simulink model "VentilatorActivity"  (R2024b)
settings: Solver=VariableStepAuto  StartTime=0.0  StopTime=10.0  RelTol=1e-3
model workspace (MAT data in the model file):
  HeatCmd = Simulink.Bus
  HeatCmd.Alignment = -1
  HeatCmd.PreserveElementDimensions = 0
  HeatCmd.Elements_internal = Simulink.BusElement
  HeatCmd.Elements_internal.DimensionsMode = 'Fixed'
  HeatCmd.Elements_internal.SamplingMode = 'Sample based'
  HeatCmd.Elements_internal.SampleTime = -1
  HeatCmd.Elements_internal.Name = 'Element'
  HeatCmd.Elements_internal.DataType_internal = 'double'
  HeatCmd.Elements_internal.Complexity = 'real'
  HeatCmd.Elements_internal.Dimensions = 1
  HeatCmd.DataScope = 'Auto'
  HeaterCmd = Simulink.Bus
  HeaterCmd.Alignment = -1
  HeaterCmd.PreserveElementDimensions = 0
  HeaterCmd.DataScope = 'Auto'
  HumidSens = Simulink.Bus
  HumidSens.Alignment = -1
  HumidSens.PreserveElementDimensions = 0
  HumidSens.DataScope = 'Auto'
  init = Simulink.Bus
  init.Alignment = -1
  init.PreserveElementDimensions = 0
  init.DataScope = 'Auto'
settings Model: Creator=ppatel  LastModifiedBy=ppatel

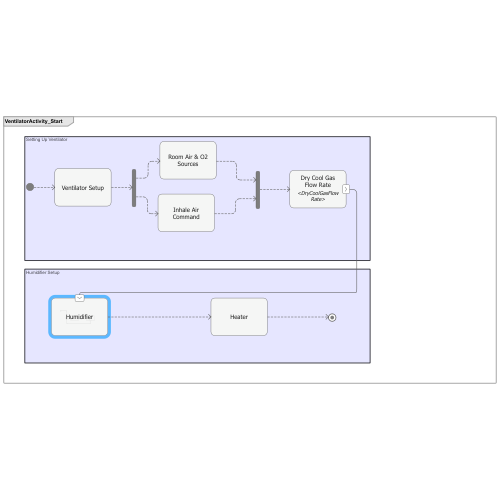
[thumbnail: Simulink's stored preview of the top-level diagram]
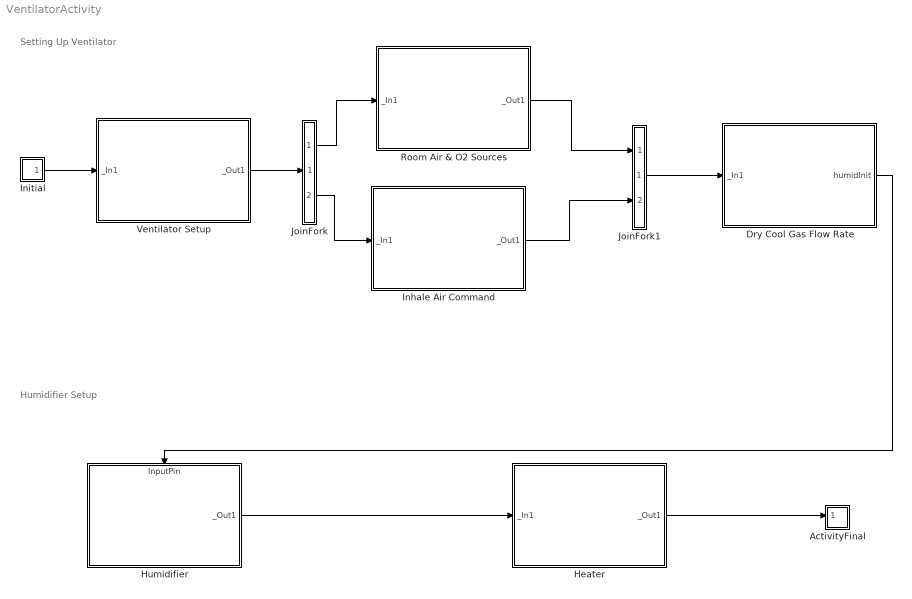
== system VentilatorActivity ==
  note: Humidifier Setup
  note: Setting Up Ventilator
  ActivityFinal : Subsystem
      settings: CopyFcn=set_param(gcbh,'LinkStatus','none');  PortSchema="{\"entries\":[{\"content\":{\"sides\":[{\"content\":{\"connectorIds\":[\"In1\"]},\"type\":\"ConnectorPlacement.EquallySpacedRectSide\",\"uuid\":\"545063dc-4e23-42d6-a986-4c8405208aa1\"},{\"content\":{\"side\":\"RIGHT\"},\"type\":\"ConnectorPlacement.EquallySpacedRectSide\",\"uuid\":\"029392fb-54d3-4ba8-8de1-0e1a97e1bcb4\"},{\"content\":{\"side\":\"TOP\"},\"type\":\"ConnectorPlacement.EquallySpacedRectSide\",\"uuid\":\"54e3c782-8e9d-4642-bf02-641c09921257\"}]},\"type\":\"ConnectorPlacement.EquallySpacedConnector\",\"uuid\":\"f1116680-de99-432f-896c-332f12d99629\"}],\"packageUris\":[\"http://schema.mathworks.com/mf0/Connector/R2020b\"],\"version\":\"1.0\"}"
  Dry Cool Gas Flow Rate : Subsystem
      settings: CopyFcn=set_param(gcbh,'LinkStatus','none');  PortSchema="{\"entries\":[{\"content\":{\"sides\":[{\"content\":{\"connectorIds\":[\"In1\"]},\"type\":\"ConnectorPlacement.EquallySpacedRectSide\",\"uuid\":\"4f1d0bb7-2a97-405d-887b-71e646284e96\"},{\"content\":{\"connectorIds\":[\"Out1\"],\"side\":\"RIGHT\"},\"type\":\"ConnectorPlacement.EquallySpacedRectSide\",\"uuid\":\"0e26442f-68e1-4c32-ac28-bf73737006e5\"},{\"content\":{\"side\":\"TOP\"},\"type\":\"ConnectorPlacement.EquallySpacedRectSide\",\"uuid\":\"07aed82e-d8ef-4f36-9f89-d56db089fe7b\"}]},\"type\":\"ConnectorPlacement.EquallySpacedConnector\",\"uuid\":\"4c88084e-95e1-4023-9a32-ff830e393fdc\"}],\"packageUris\":[\"http://schema.mathworks.com/mf0/Connector/R2020b\"],\"version\":\"1.0\"}"
  Heater : Subsystem
      settings: CopyFcn=set_param(gcbh,'LinkStatus','none');  PortSchema="{\"entries\":[{\"content\":{\"sides\":[{\"content\":{\"connectorIds\":[\"In1\"]},\"type\":\"ConnectorPlacement.EquallySpacedRectSide\",\"uuid\":\"da638e69-4a2c-4548-ace4-820cc1f60a8d\"},{\"content\":{\"connectorIds\":[\"Out1\"],\"side\":\"RIGHT\"},\"type\":\"ConnectorPlacement.EquallySpacedRectSide\",\"uuid\":\"6a8a70e9-7f6e-4f36-a19f-a4054ca44662\"},{\"content\":{\"side\":\"TOP\"},\"type\":\"ConnectorPlacement.EquallySpacedRectSide\",\"uuid\":\"d1e931e2-f76e-4992-8014-0092805a8671\"}]},\"type\":\"ConnectorPlacement.EquallySpacedConnector\",\"uuid\":\"55c0ca13-68f0-475a-9ea9-fab942dd6d78\"}],\"packageUris\":[\"http://schema.mathworks.com/mf0/Connector/R2020b\"],\"version\":\"1.0\"}"
  Humidifier : Subsystem
      settings: CopyFcn=set_param(gcbh,'LinkStatus','none');  PortSchema="{\"entries\":[{\"content\":{\"sides\":[{\"content\":{},\"type\":\"ConnectorPlacement.EquallySpacedRectSide\",\"uuid\":\"da638e69-4a2c-4548-ace4-820cc1f60a8d\"},{\"content\":{\"connectorIds\":[\"Out1\"],\"side\":\"RIGHT\"},\"type\":\"ConnectorPlacement.EquallySpacedRectSide\",\"uuid\":\"6a8a70e9-7f6e-4f36-a19f-a4054ca44662\"},{\"content\":{\"connectorIds\":[\"In1\"],\"side\":\"TOP\"},\"type\":\"ConnectorPlacement.EquallySpacedRectSide\",\"uuid\":\"d1e931e2-f76e-4992-8014-0092805a8671\"}]},\"type\":\"ConnectorPlacement.EquallySpacedConnector\",\"uuid\":\"55c0ca13-68f0-475a-9ea9-fab942dd6d78\"}],\"packageUris\":[\"http://schema.mathworks.com/mf0/Connector/R2020b\"],\"version\":\"1.0\"}"
  Inhale Air Command : Subsystem
      settings: CopyFcn=set_param(gcbh,'LinkStatus','none');  PortSchema="{\"entries\":[{\"content\":{\"sides\":[{\"content\":{\"connectorIds\":[\"In1\"]},\"type\":\"ConnectorPlacement.EquallySpacedRectSide\",\"uuid\":\"da638e69-4a2c-4548-ace4-820cc1f60a8d\"},{\"content\":{\"connectorIds\":[\"Out1\"],\"side\":\"RIGHT\"},\"type\":\"ConnectorPlacement.EquallySpacedRectSide\",\"uuid\":\"6a8a70e9-7f6e-4f36-a19f-a4054ca44662\"},{\"content\":{\"side\":\"TOP\"},\"type\":\"ConnectorPlacement.EquallySpacedRectSide\",\"uuid\":\"d1e931e2-f76e-4992-8014-0092805a8671\"}]},\"type\":\"ConnectorPlacement.EquallySpacedConnector\",\"uuid\":\"55c0ca13-68f0-475a-9ea9-fab942dd6d78\"}],\"packageUris\":[\"http://schema.mathworks.com/mf0/Connector/R2020b\"],\"version\":\"1.0\"}"
  Initial : Subsystem
      settings: CopyFcn=set_param(gcbh,'LinkStatus','none');  PortSchema="{\"entries\":[{\"content\":{\"sides\":[{\"content\":{},\"type\":\"ConnectorPlacement.EquallySpacedRectSide\",\"uuid\":\"da638e69-4a2c-4548-ace4-820cc1f60a8d\"},{\"content\":{\"connectorIds\":[\"Out1\"],\"side\":\"RIGHT\"},\"type\":\"ConnectorPlacement.EquallySpacedRectSide\",\"uuid\":\"6a8a70e9-7f6e-4f36-a19f-a4054ca44662\"},{\"content\":{\"side\":\"TOP\"},\"type\":\"ConnectorPlacement.EquallySpacedRectSide\",\"uuid\":\"d1e931e2-f76e-4992-8014-0092805a8671\"}]},\"type\":\"ConnectorPlacement.EquallySpacedConnector\",\"uuid\":\"55c0ca13-68f0-475a-9ea9-fab942dd6d78\"}],\"packageUris\":[\"http://schema.mathworks.com/mf0/Connector/R2020b\"],\"version\":\"1.0\"}"
  JoinFork : Subsystem
      settings: CopyFcn=set_param(gcbh,'LinkStatus','none');  PortSchema="{\"entries\":[{\"content\":{\"sides\":[{\"content\":{\"connectorIds\":[\"In1\"]},\"type\":\"ConnectorPlacement.EquallySpacedRectSide\",\"uuid\":\"da638e69-4a2c-4548-ace4-820cc1f60a8d\"},{\"content\":{\"connectorIds\":[\"Out1\",\"Out2\"],\"side\":\"RIGHT\"},\"type\":\"ConnectorPlacement.EquallySpacedRectSide\",\"uuid\":\"6a8a70e9-7f6e-4f36-a19f-a4054ca44662\"},{\"content\":{\"side\":\"TOP\"},\"type\":\"ConnectorPlacement.EquallySpacedRectSide\",\"uuid\":\"d1e931e2-f76e-4992-8014-0092805a8671\"}]},\"type\":\"ConnectorPlacement.EquallySpacedConnector\",\"uuid\":\"55c0ca13-68f0-475a-9ea9-fab942dd6d78\"}],\"packageUris\":[\"http://schema.mathworks.com/mf0/Connector/R2020b\"],\"version\":\"1.0\"}"
  JoinFork1 : Subsystem
      settings: CopyFcn=set_param(gcbh,'LinkStatus','none');  PortSchema="{\"entries\":[{\"content\":{\"sides\":[{\"content\":{\"connectorIds\":[\"In1\",\"In2\"]},\"type\":\"ConnectorPlacement.EquallySpacedRectSide\",\"uuid\":\"da638e69-4a2c-4548-ace4-820cc1f60a8d\"},{\"content\":{\"connectorIds\":[\"Out1\"],\"side\":\"RIGHT\"},\"type\":\"ConnectorPlacement.EquallySpacedRectSide\",\"uuid\":\"6a8a70e9-7f6e-4f36-a19f-a4054ca44662\"},{\"content\":{\"side\":\"TOP\"},\"type\":\"ConnectorPlacement.EquallySpacedRectSide\",\"uuid\":\"d1e931e2-f76e-4992-8014-0092805a8671\"}]},\"type\":\"ConnectorPlacement.EquallySpacedConnector\",\"uuid\":\"55c0ca13-68f0-475a-9ea9-fab942dd6d78\"}],\"packageUris\":[\"http://schema.mathworks.com/mf0/Connector/R2020b\"],\"version\":\"1.0\"}"
  Room Air & O2 Sources : Subsystem
      settings: CopyFcn=set_param(gcbh,'LinkStatus','none');  PortSchema="{\"entries\":[{\"content\":{\"sides\":[{\"content\":{\"connectorIds\":[\"In1\"]},\"type\":\"ConnectorPlacement.EquallySpacedRectSide\",\"uuid\":\"da638e69-4a2c-4548-ace4-820cc1f60a8d\"},{\"content\":{\"connectorIds\":[\"Out1\"],\"side\":\"RIGHT\"},\"type\":\"ConnectorPlacement.EquallySpacedRectSide\",\"uuid\":\"6a8a70e9-7f6e-4f36-a19f-a4054ca44662\"},{\"content\":{\"side\":\"TOP\"},\"type\":\"ConnectorPlacement.EquallySpacedRectSide\",\"uuid\":\"d1e931e2-f76e-4992-8014-0092805a8671\"}]},\"type\":\"ConnectorPlacement.EquallySpacedConnector\",\"uuid\":\"55c0ca13-68f0-475a-9ea9-fab942dd6d78\"}],\"packageUris\":[\"http://schema.mathworks.com/mf0/Connector/R2020b\"],\"version\":\"1.0\"}"
  Ventilator Setup : Subsystem
      settings: CopyFcn=set_param(gcbh,'LinkStatus','none');  PortSchema="{\"entries\":[{\"content\":{\"sides\":[{\"content\":{\"connectorIds\":[\"In1\"]},\"type\":\"ConnectorPlacement.EquallySpacedRectSide\",\"uuid\":\"da638e69-4a2c-4548-ace4-820cc1f60a8d\"},{\"content\":{\"connectorIds\":[\"Out1\"],\"side\":\"RIGHT\"},\"type\":\"ConnectorPlacement.EquallySpacedRectSide\",\"uuid\":\"6a8a70e9-7f6e-4f36-a19f-a4054ca44662\"},{\"content\":{\"side\":\"TOP\"},\"type\":\"ConnectorPlacement.EquallySpacedRectSide\",\"uuid\":\"d1e931e2-f76e-4992-8014-0092805a8671\"}]},\"type\":\"ConnectorPlacement.EquallySpacedConnector\",\"uuid\":\"55c0ca13-68f0-475a-9ea9-fab942dd6d78\"}],\"packageUris\":[\"http://schema.mathworks.com/mf0/Connector/R2020b\"],\"version\":\"1.0\"}"
  wires:
  Room Air & O2 Sources/1(_Out1) -> JoinFork1/1(_In1)
  Ventilator Setup/1(_Out1) -> JoinFork/1(_In1)
  JoinFork1/1(_Out1) -> Dry Cool Gas Flow Rate/1(_In1)
  JoinFork/2(_Out2) -> Inhale Air Command/1(_In1)
  Initial/1(_Out1) -> Ventilator Setup/1(_In1)
  Inhale Air Command/1(_Out1) -> JoinFork1/2(_In2)
  JoinFork/1(_Out1) -> Room Air & O2 Sources/1(_In1)
  Dry Cool Gas Flow Rate/1(humidInit) -> Humidifier/1(InputPin)
  Heater/1(_Out1) -> ActivityFinal/1(_In1)
  Humidifier/1(_Out1) -> Heater/1(_In1)

== system VentilatorActivity/ActivityFinal ==
  _In1 : Inport

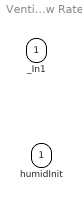
== system VentilatorActivity/Dry Cool Gas Flow Rate ==
  _In1 : Inport
  humidInit : Outport  PortDimensions=1

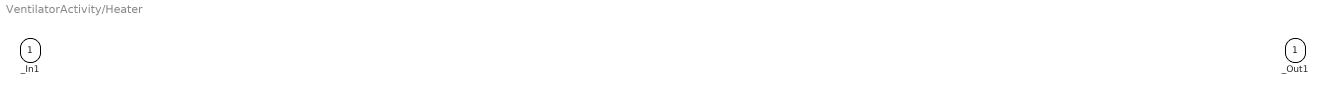
== system VentilatorActivity/Heater ==
  _In1 : Inport
  _Out1 : Outport

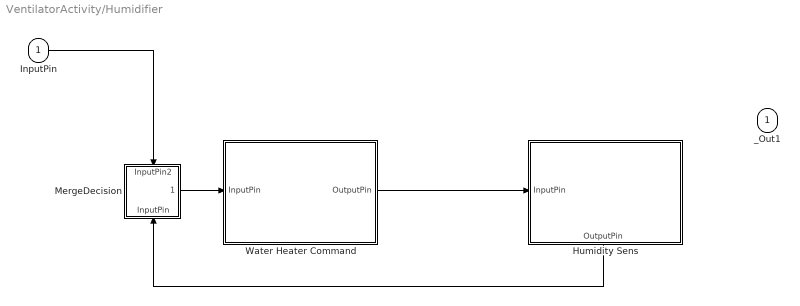
== system VentilatorActivity/Humidifier ==
  InputPin : Inport
  Humidity Sens : Subsystem
      settings: CopyFcn=set_param(gcbh,'LinkStatus','none');  PortSchema="{\"entries\":[{\"content\":{\"sides\":[{\"content\":{\"connectorIds\":[\"In1\"]},\"type\":\"ConnectorPlacement.EquallySpacedRectSide\",\"uuid\":\"da638e69-4a2c-4548-ace4-820cc1f60a8d\"},{\"content\":{\"side\":\"RIGHT\"},\"type\":\"ConnectorPlacement.EquallySpacedRectSide\",\"uuid\":\"6a8a70e9-7f6e-4f36-a19f-a4054ca44662\"},{\"content\":{\"side\":\"TOP\"},\"type\":\"ConnectorPlacement.EquallySpacedRectSide\",\"uuid\":\"d1e931e2-f76e-4992-8014-0092805a8671\"},{\"content\":{\"connectorIds\":[\"Out1\"],\"side\":\"BOTTOM\"},\"type\":\"ConnectorPlacement.EquallySpacedRectSide\",\"uuid\":\"10984552-7b35-4f88-a27c-5daa08678015\"}]},\"type\":\"ConnectorPlacement.EquallySpacedConnector\",\"uuid\":\"55c0ca13-68f0-475a-9ea9-fab942dd6d78\"}],\"packageUris\":[\"http://schema.mathworks.com/mf0/Connector/R2020b\"],\"version\":\"1.0\"}"
  MergeDecision : Subsystem
      settings: CopyFcn=set_param(gcbh,'LinkStatus','none');  PortSchema="{\"entries\":[{\"content\":{\"sides\":[{\"content\":{},\"type\":\"ConnectorPlacement.EquallySpacedRectSide\",\"uuid\":\"da638e69-4a2c-4548-ace4-820cc1f60a8d\"},{\"content\":{\"connectorIds\":[\"Out1\"],\"side\":\"RIGHT\"},\"type\":\"ConnectorPlacement.EquallySpacedRectSide\",\"uuid\":\"6a8a70e9-7f6e-4f36-a19f-a4054ca44662\"},{\"content\":{\"connectorIds\":[\"In2\"],\"side\":\"TOP\"},\"type\":\"ConnectorPlacement.EquallySpacedRectSide\",\"uuid\":\"d1e931e2-f76e-4992-8014-0092805a8671\"},{\"content\":{\"connectorIds\":[\"In1\"],\"side\":\"BOTTOM\"},\"type\":\"ConnectorPlacement.EquallySpacedRectSide\",\"uuid\":\"1d127de0-f1c8-411a-9d19-34e7d29db091\"}]},\"type\":\"ConnectorPlacement.EquallySpacedConnector\",\"uuid\":\"55c0ca13-68f0-475a-9ea9-fab942dd6d78\"}],\"packageUris\":[\"http://schema.mathworks.com/mf0/Connector/R2020b\"],\"version\":\"1.0\"}"
  Water Heater Command : Subsystem
      settings: CopyFcn=set_param(gcbh,'LinkStatus','none');  PortSchema="{\"entries\":[{\"content\":{\"sides\":[{\"content\":{\"connectorIds\":[\"In1\"]},\"type\":\"ConnectorPlacement.EquallySpacedRectSide\",\"uuid\":\"da638e69-4a2c-4548-ace4-820cc1f60a8d\"},{\"content\":{\"connectorIds\":[\"Out1\"],\"side\":\"RIGHT\"},\"type\":\"ConnectorPlacement.EquallySpacedRectSide\",\"uuid\":\"6a8a70e9-7f6e-4f36-a19f-a4054ca44662\"},{\"content\":{\"side\":\"TOP\"},\"type\":\"ConnectorPlacement.EquallySpacedRectSide\",\"uuid\":\"d1e931e2-f76e-4992-8014-0092805a8671\"},{\"content\":{\"side\":\"BOTTOM\"},\"type\":\"ConnectorPlacement.EquallySpacedRectSide\",\"uuid\":\"c8c6cd51-bc28-4508-8599-fc70c851359e\"}]},\"type\":\"ConnectorPlacement.EquallySpacedConnector\",\"uuid\":\"55c0ca13-68f0-475a-9ea9-fab942dd6d78\"}],\"packageUris\":[\"http://schema.mathworks.com/mf0/Connector/R2020b\"],\"version\":\"1.0\"}"
  _Out1 : Outport
  wires:
  Water Heater Command/1(OutputPin) -> Humidity Sens/1(InputPin)
  MergeDecision/1(_Out1) -> Water Heater Command/1(InputPin)
  InputPin/1 -> MergeDecision/2(InputPin2)
  Humidity Sens/1(OutputPin) -> MergeDecision/1(InputPin)

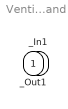
== system VentilatorActivity/Inhale Air Command ==
  _In1 : Inport
  _Out1 : Outport

== system VentilatorActivity/Initial ==
  _Out1 : Outport

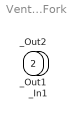
== system VentilatorActivity/JoinFork ==
  _In1 : Inport
  _Out1 : Outport
  _Out2 : Outport  Port=2

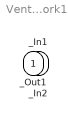
== system VentilatorActivity/JoinFork1 ==
  _In1 : Inport
  _In2 : Inport  Port=2
  _Out1 : Outport

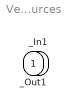
== system VentilatorActivity/Room Air & O2 Sources ==
  _In1 : Inport
  _Out1 : Outport

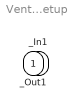
== system VentilatorActivity/Ventilator Setup ==
  _In1 : Inport
  _Out1 : Outport

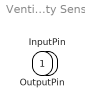
== system VentilatorActivity/Humidifier/Humidity Sens ==
  InputPin : Inport
  OutputPin : Outport  OutDataTypeStr=double  PortDimensions=1

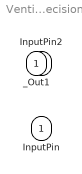
== system VentilatorActivity/Humidifier/MergeDecision ==
  InputPin : Inport
  InputPin2 : Inport  Port=2
  _Out1 : Outport

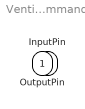
== system VentilatorActivity/Humidifier/Water Heater Command ==
  InputPin : Inport
  OutputPin : Outport  OutDataTypeStr=double  PortDimensions=1
